simulink model "model_v2"  (R2017a)
settings: Solver=VariableStepAuto  StartTime=0.0  StopTime=10  FixedStep=Ts  RelTol=1e-4  EnableMultiTasking=on
model workspace (MAT data in the model file):
  I1 = 0.0029
  I2 = 7.8856e-05
  L1 = 1
  L2 = 1.1
  P1 = 0.0036
  P2 = 0.000258856
  P3 = 0.0003
  Ts = 0.01
  b1 = 5.8039
  b2 = 3.125e-05
  c1 = -0.04
  c2 = 0.06
  g = 9.81
  g1 = 8.50881864967e-18
  g2 = 0.02943
  h = 0.01
  initial_state = [0 0]
  k_m = 41.0587
  l1 = 0.1
  l2 = 0.1
  m1 = 0.125
  m2 = 0.05
  par = [0.0036; 0.000258856; 0.0003; 8.50881864967e-18; 0.02943]
  sim_time = 10
  tau_e = 0.0312
  torque = 0
  torque_bypass = 0
settings Model: Creator=Nathan  LastModifiedBy=Ortix
settings DataIOCC: InitialState=states  LimitDataPoints=on  SaveFormat=Array
settings OptimizationCC: LifeSpan=inf
settings DebuggingCC: AllowSymbolicDim=off  SFUnexpectedBacktrackingDiag=warning  SFNoUnconditionalDefaultTransitionDiag=warning  SFExecutionAtInitializationDiag=none
settings HardwareCC: ProdBitPerPointer=32  ProdBitPerSizeT=32  ProdBitPerPtrDiffT=32  ProdLargestAtomicFloat=None  ProdIntDivRoundTo=Undefined  ProdEndianess=Unspecified  ProdWordSize=32  ProdHWDeviceType=32-bit Generic
settings ModelReferenceCC: PropagateSignalLabelsOutOfModel=off
settings GRTTargetCC: TargetLangStandard=C89/C90 (ANSI)  GeneratePreprocessorConditionals=Disable all
settings ConfigComp: CovMetricSettings=dw  CovHtmlReporting=on  CovSaveCumulativeToWorkspaceVar=on  CovSaveSingleToWorkspaceVar=on  CovExternalEMLEnable=off

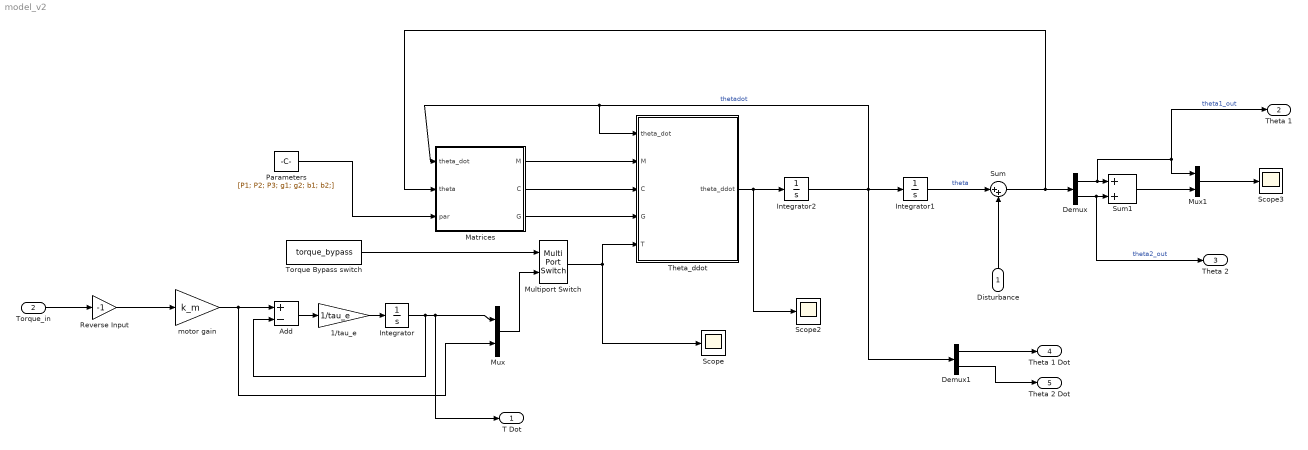
== system model_v2 ==
  Disturbance : Inport  PortDimensions=2
  Torque_in : Inport  Port=2
  "1/tau_e " : Gain  Gain=1/tau_e
  Add : Sum  Inputs=+-
  Demux : Demux  Outputs=2
  Demux1 : Demux  Outputs=2
  Integrator : Integrator
  Integrator1 : Integrator  InitialCondition=initial_state
  Integrator2 : Integrator
  Matrices : MATLAB Function  TreatAsAtomicUnit=on
  Multiport Switch : MultiPortSwitch  DataPortOrder=Zero-based contiguous  Inputs=1
  Mux : Mux  Inputs=2
  Mux1 : Mux  Inputs=2
  Parameters : Constant  Value=|
      | [P1; P2; P3; g1;
      | g2;
      | b1;
      | b2;]
  Reverse Input : Gain  Gain=-1
  Scope : Scope
  Scope2 : Scope
  Scope3 : Scope
  Sum : Sum  Inputs=|++
  Sum1 : Sum
  "Theta_ddot " : MATLAB Function  TreatAsAtomicUnit=on
  Torque Bypass switch : Constant  Value=torque_bypass
  "motor gain " : Gain  Gain=k_m
  T Dot : Outport
  Theta 1 : Outport  Port=2
  Theta 2 : Outport  Port=3
  Theta 1 Dot : Outport  Port=4
  Theta 2 Dot : Outport  Port=5
  wires:
  Torque_in/1 -> Reverse Input/1
  Integrator/1 -> Add/2, T Dot/1, Mux/1
  Integrator2/1 -> Integrator1/1, Demux1/1, "Theta_ddot "/1(theta_dot), Matrices/1(theta_dot)  "thetadot"
  Matrices/3(G) -> "Theta_ddot "/4(G)
  Matrices/1(M) -> "Theta_ddot "/2(M)
  "Theta_ddot "/1(theta_ddot) -> Integrator2/1, Scope2/1
  Matrices/2(C) -> "Theta_ddot "/3(C)
  Add/1 -> "1/tau_e "/1
  "1/tau_e "/1 -> Integrator/1
  Integrator1/1 -> Sum/1  "theta"
  Mux/1 -> Multiport Switch/2
  Torque Bypass switch/1 -> Multiport Switch/1
  "motor gain "/1 -> Mux/2, Add/1
  Demux/1 -> Theta 1/1, Mux1/1, Sum1/1  "theta1_out"
  Demux/2 -> Theta 2/1, Sum1/2  "theta2_out"
  Reverse Input/1 -> "motor gain "/1
  Sum1/1 -> Mux1/2
  Sum/1 -> Matrices/2(theta), Demux/1
  Mux1/1 -> Scope3/1
  Multiport Switch/1 -> Scope/1, "Theta_ddot "/5(T)
  Disturbance/1 -> Sum/2
  Demux1/1 -> Theta 1 Dot/1
  Demux1/2 -> Theta 2 Dot/1
  Parameters/1 -> Matrices/3(par)

== matlab function model_v2/Theta_ddot  ==
  data: theta_dot input; M input; C input; G input; theta_ddot output; T input
function theta_ddot = fcn(theta_dot,M,C,G,T)
theta_ddot = [0;0];

theta_ddot = M\[T;0] - M\C*theta_dot - M\G;

== matlab function model_v2/Matrices ==
  data: theta_dot input; theta input; M output; C output; G output; par input size=[7;1]
function [M, C, G] = fcn(theta_dot, theta, par)

M = zeros(2);
C = zeros(2);
G = [0;0];


P1 = par(1);
P2 = par(2);
P3 = par(3);
g1 = par(4);
g2 = par(5);
b1 = par(6);
b2 = par(7);

M = [(P1 + P2 + 2*P3*cos(theta(2)))               (P2 + P3*cos(theta(2))) ;
     (P2 + P3*cos(theta(2)))                       P2                   ];
 
 
C = [(b1 - P3*theta_dot(2)*sin(theta(2)))           (-P3*(theta_dot(1)+theta_dot(2))*sin(theta(2))) ;
     (P3*theta_dot(1)*sin(theta(2)))                 b2                                      ];
     
G = [(-g1*sin(theta(1))-g2*sin(theta(1) + theta(2))) ;
      -g2*sin(theta(1)+theta(2))                   ];
% function [M, C, G] = fcn(theta_dot, theta, par)
% 
% M = zeros(2);
% C = zeros(2);
% G = [0;0];
% 
% 
% M = [(par.P1 + par.P2 + 2*par.P3*cos(theta(2))) (par.P2 + par.P3*cos(theta(2))) ;
%     (par.P2 + par.P3*cos(theta(2)))                       par.P2               ];
% 
% 
% C = [(par.b1 - par.P3*theta_dot(2)*sin(theta(2))) (-par.P3*(theta_dot(1)+theta_dot(2))*sin(theta(2))) ;
%     (par.P3*theta_dot(1)*sin(theta(2)))                 par.b2          ];
% 
% G = [(-par.g1*sin(theta(1))-par.g2*sin(theta(1) + theta(2))) ;
%     -par.g2*sin(theta(1)+theta(2))                   ];
